simulink model "Astrini_YuNonLinearTissueWithStatesWithNoise"  (Simulink 8.3)
settings: Solver=ode3  StartTime=0.0  StopTime=tend  FixedStep=1e-3  MaxStep=0.1  RelTol=1e-3
values from neighbouring files (symbols this model uses):
  A = 2    [SimData.m]    (also in SimDataPrelim_NL.m = 100)
  alphaYu = alphaSi(actualIndex)    [SimData.m]
  betaYu = betaSi(actualIndex)    [SimData.m]
  dYu = dSi(actualIndex)    [SimData.m]
  Fgrasp = 2    [SimData.m]
  mYu = .005    (= 0.005)    [SimData.m]
settings Model: Creator=pjseiler  LastModifiedBy=timk
settings OptimizationCC: ExpressionDepthLimit=2147483647
settings DebuggingCC: MultiTaskDSMMsg=warning  MultiTaskCondExecSysMsg=none  FcnCallInpInsideContextMsg=UseLocalSettings
settings RTWCC: IncludeERTFirstTime=on

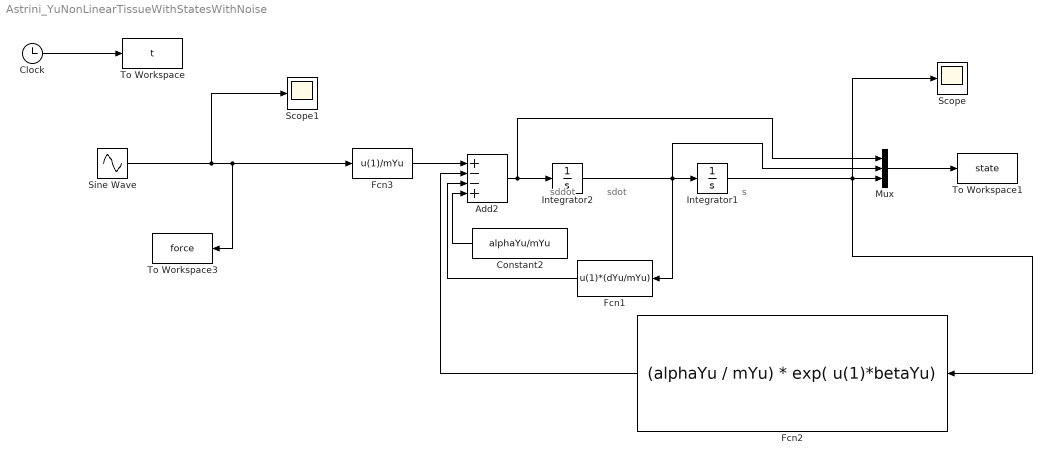
== system Astrini_YuNonLinearTissueWithStatesWithNoise ==
  note: sddot
  note: sdot
  note: s
  Add2 : Sum  Inputs=+--+
  Clock : Clock
  Constant2 : Constant  Value=alphaYu/mYu
  Fcn1 : Fcn  Expr=u(1)*(dYu/mYu)
  Fcn2 : Fcn  Expr=(alphaYu / mYu) * exp( u(1)*betaYu)
  Fcn3 : Fcn  Expr=u(1)/mYu
  Integrator1 : Integrator
  Integrator2 : Integrator
  Mux : Mux  Inputs=3
  Scope : Scope
  Scope1 : Scope
  Sine Wave : Sin  Amplitude=A/2  Bias=A/2  Frequency=Fgrasp*(2*pi)  Phase=-pi/2  SampleTime=0
  To Workspace : ToWorkspace  VariableName=t  SampleTime=-1
  To Workspace1 : ToWorkspace  VariableName=state  SampleTime=-1
  To Workspace3 : ToWorkspace  VariableName=force  SampleTime=-1
  wires:
  Clock/1 -> To Workspace/1
  Integrator2/1 -> Fcn1/1, Integrator1/1, Mux/2
  Integrator1/1 -> Fcn2/1, Scope/1, Mux/3
  Constant2/1 -> Add2/4
  Add2/1 -> Integrator2/1, Mux/1
  Fcn1/1 -> Add2/3
  Fcn2/1 -> Add2/2
  Fcn3/1 -> Add2/1
  Mux/1 -> To Workspace1/1
  Sine Wave/1 -> Scope1/1, Fcn3/1, To Workspace3/1
